simulink model "Modelo_nolineal_5GDL_COMPLETO_2022"  (R2021b)
settings: Solver=VariableStepAuto  StartTime=0.0  StopTime=5  FixedStep=T  RelTol=1e-3
values from neighbouring files (symbols this model uses):
  g = 9.81    [main.m]
undefined symbols (not defined in the file or in its folder): AG0, k1, k2, k3, l1, l2, l3, p1, p2, pod, ROTX_0, ROTY_0, ROTZ_0, y_ini, z_ini
settings Model: Creator=EDMAOR  LastModifiedBy=emate
settings SolverCC: AlgebraicLoopSolver=TrustRegion
settings DebuggingCC: SFMachineParentedDataDiag=warning
settings SFSimCC: CustomCodeUndefinedFunction=UseInterfaceOnly

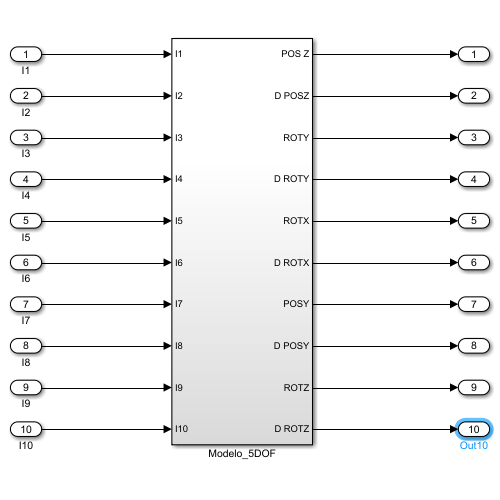
[thumbnail: Simulink's stored preview of the top-level diagram]
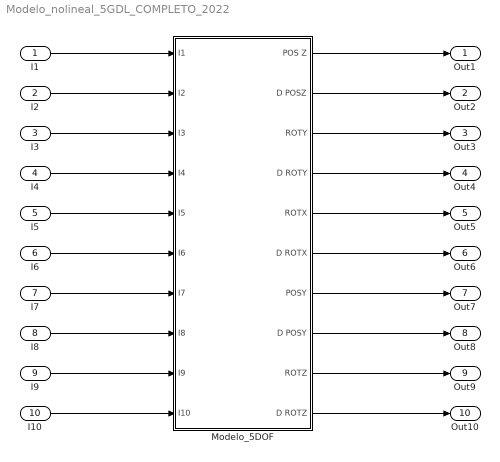
== system Modelo_nolineal_5GDL_COMPLETO_2022 ==
  I1 : Inport
  I2 : Inport  Port=2
  I3 : Inport  Port=3
  I4 : Inport  Port=4
  I5 : Inport  Port=5
  I6 : Inport  Port=6
  I7 : Inport  Port=7
  I8 : Inport  Port=8
  I9 : Inport  Port=9
  I10 : Inport  Port=10
  Modelo_5DOF : Subsystem
  Out1 : Outport
  Out2 : Outport  Port=2
  Out3 : Outport  Port=3
  Out4 : Outport  Port=4
  Out5 : Outport  Port=5
  Out6 : Outport  Port=6
  Out7 : Outport  Port=7
  Out8 : Outport  Port=8
  Out9 : Outport  Port=9
  Out10 : Outport  Port=10
  wires:
  Modelo_5DOF/1(POS Z) -> Out1/1
  I1/1 -> Modelo_5DOF/1(I1)
  I2/1 -> Modelo_5DOF/2(I2)
  I3/1 -> Modelo_5DOF/3(I3)
  I4/1 -> Modelo_5DOF/4(I4)
  I5/1 -> Modelo_5DOF/5(I5)
  I6/1 -> Modelo_5DOF/6(I6)
  Modelo_5DOF/2(D POSZ) -> Out2/1
  Modelo_5DOF/3(ROTY) -> Out3/1
  Modelo_5DOF/4(D ROTY) -> Out4/1
  Modelo_5DOF/5(ROTX) -> Out5/1
  Modelo_5DOF/6(D ROTX) -> Out6/1
  I7/1 -> Modelo_5DOF/7(I7)
  I8/1 -> Modelo_5DOF/8(I8)
  I9/1 -> Modelo_5DOF/9(I9)
  I10/1 -> Modelo_5DOF/10(I10)
  Modelo_5DOF/7(POSY) -> Out7/1
  Modelo_5DOF/8(D POSY) -> Out8/1
  Modelo_5DOF/9(ROTZ) -> Out9/1
  Modelo_5DOF/10(D ROTZ) -> Out10/1

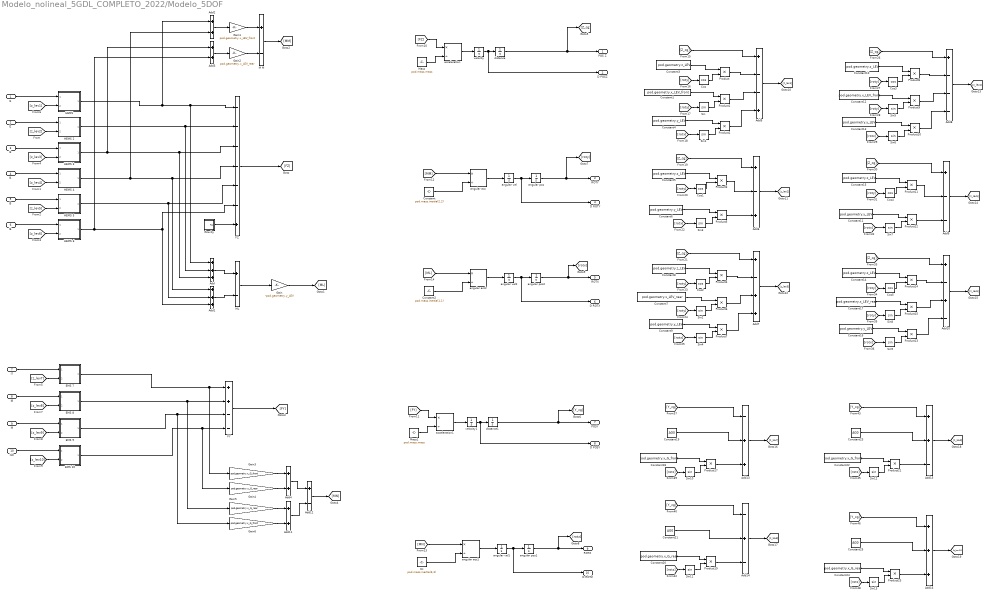
== system Modelo_nolineal_5GDL_COMPLETO_2022/Modelo_5DOF ==
  I1 : Inport
  I2 : Inport  Port=2
  I3 : Inport  Port=3
  I4 : Inport  Port=4
  I5 : Inport  Port=5
  I6 : Inport  Port=6
  I7 : Inport  Port=7
  I8 : Inport  Port=8
  I9 : Inport  Port=9
  I10 : Inport  Port=10
  Add : Sum  Inputs=+++
  Add1 : Sum  Inputs=+++
  Add10 : Sum  Inputs=+-+-
  Add{2..4,11} (4 alike) : Sum
  Add12 : Sum  Inputs=+-
  Add13 : Sum  Inputs=-++
  Add14 : Sum  Inputs=-+-
  Add15 : Sum  Inputs=++-
  Add16 : Sum  Inputs=+++
  Add5 : Sum  Inputs=+--+
  Add6 : Sum  Inputs=+-+
  Add7 : Sum  Inputs=+-++
  Add8 : Sum  Inputs=+---
  Add9 : Sum  Inputs=+--
  Constant : Constant  Value=pod.mass.inertia(2,2)
  Constant1 : Constant  Value=pod.geometry.x_LEV_front
  Constant{3,5,8,10,14..15} (6 alike) : Constant  Value=pod.geometry.z_LEV
  Constant{4,6,9,11,13,16} (6 alike) : Constant  Value=pod.geometry.y_LEV
  Constant12 : Constant  Value=pod.geometry.x_LEV_front
  Constant17 : Constant  Value=pod.geometry.x_LEV_rear
  Constant18 : Constant  Value=pod.geometry.x_G_front
  Constant{19,21,23,25} (4 alike) : Constant  Value=AG0
  Constant2 : Constant  Value=pod.mass.inertia(1,1)
  Constant20 : Constant  Value=pod.geometry.x_G_rear
  Constant22 : Constant  Value=pod.geometry.x_G_front
  Constant24 : Constant  Value=pod.geometry.x_G_rear
  Constant7 : Constant  Value=pod.geometry.x_LEV_rear
  Cos{,1..5} (6 alike) : Trigonometry  Operator=cos
  EMS 10 : Subsystem
  EMS 7 : Subsystem
  EMS 8 : Subsystem
  EMS 9 : Subsystem
  FY : Sum  Inputs=++--
  FZ : Sum  Inputs=------+
  Gain : Gain  Gain=-pod.geometry.y_LEV
  Gain1 : Gain  Gain=pod.geometry.x_LEV_front
  Gain2 : Gain  Gain=pod.geometry.x_LEV_rear
  Gain3 : Gain  Gain=pod.geometry.x_G_front
  Gain4 : Gain  Gain=pod.geometry.x_G_rear
  Gain5 : Gain  Gain=pod.geometry.x_G_rear
  Gain6 : Gain  Gain=pod.geometry.x_G_front
  Gravity : Subsystem
  "HEMS " : Subsystem
  HEMS 2 : Subsystem
  HEMS 3 : Subsystem
  HEMS 4 : Subsystem
  HEMS 5 : Subsystem
  HEMS 6 : Subsystem
  Izz : Constant  Value=pod.mass.inertia(3,3)
  M M : Sum  Inputs=+-
  ML : Sum  Inputs=+-
  Mass : Constant  Value=pod.mass.mass
  Mass1 : Constant  Value=pod.mass.mass
  Product{,1..15,17,19,21,23} (20 alike) : Product
  Sin{,1..13} (14 alike) : Trigonometry
  acceleration : Product  Inputs=*/
  acceleration1 : Product  Inputs=*/
  angular acc : Product  Inputs=*/
  angular acc1 : Product  Inputs=*/
  angular acc2 : Product  Inputs=*/
  angular pos : Integrator  InitialCondition=ROTY_0
  angular pos1 : Integrator  InitialCondition=ROTZ_0
  angular pos2 : Integrator  InitialCondition=ROTX_0
  angular vel : Integrator
  angular vel1 : Integrator
  angular vel2 : Integrator
  distance : Integrator  InitialCondition=z_ini
  distance1 : Integrator  InitialCondition=y_ini
  velocity : Integrator
  velocity1 : Integrator
  POS Z : Outport  VectorParamsAs1DForOutWhenUnconnected=off
  D POSZ : Outport  Port=2  VectorParamsAs1DForOutWhenUnconnected=off
  ROTY : Outport  Port=3  VectorParamsAs1DForOutWhenUnconnected=off
  D ROTY : Outport  Port=4  VectorParamsAs1DForOutWhenUnconnected=off
  ROTX : Outport  Port=5  VectorParamsAs1DForOutWhenUnconnected=off
  D ROTX : Outport  Port=6  VectorParamsAs1DForOutWhenUnconnected=off
  POSY : Outport  Port=7  VectorParamsAs1DForOutWhenUnconnected=off
  D POSY : Outport  Port=8  VectorParamsAs1DForOutWhenUnconnected=off
  ROTZ : Outport  Port=9  VectorParamsAs1DForOutWhenUnconnected=off
  D ROTZ : Outport  Port=10  VectorParamsAs1DForOutWhenUnconnected=off
  wires:
  acceleration/1 -> velocity/1
  velocity/1 -> D POSZ/1, distance/1
  distance/1 -> [Z_cg], POS Z/1
  I1/1 -> "HEMS "/1(current 1)
  I2/1 -> HEMS 2/1(current 2)
  I3/1 -> HEMS 3/1(current 3)
  "HEMS "/1(HEMS 1) -> Add/1, FZ/1, Add2/1
  HEMS 2/1(HEMS 2) -> Add/2, FZ/2
  HEMS 3/1(HEMS 3) -> Add/3, FZ/3, Add3/1
  Mass/1 -> acceleration/2
  [z_lev2] -> HEMS 2/2(distance 2)
  [z_lev3] -> HEMS 3/2(distance 3)
  [z_lev1] -> "HEMS "/2(distance 1)
  I4/1 -> HEMS 4/1(current 4)
  I5/1 -> HEMS 5/1(current 5)
  I6/1 -> HEMS 6/1(current 6)
  [z_lev4] -> HEMS 4/2(distance 4)
  [z_lev5] -> HEMS 5/2(distance 5)
  [z_lev6] -> HEMS 6/2(distance 6)
  HEMS 4/1(HEMS 4) -> Add1/1, FZ/4, Add2/2
  HEMS 5/1(HEMS 5) -> Add1/2, FZ/5
  HEMS 6/1(HEMS 6) -> Add1/3, FZ/6, Add3/2
  Gravity/1(Fg) -> FZ/7
  FZ/1 -> [FZ]
  ML/1 -> Gain/1
  Add1/1 -> ML/2
  Add/1 -> ML/1
  M M/1 -> [MM]
  Add2/1 -> Gain1/1
  Add3/1 -> Gain2/1
  Gain/1 -> [ML]
  [FZ] -> acceleration/1
  angular vel/1 -> D ROTY/1, angular pos/1
  angular pos/1 -> [roty], ROTY/1
  angular acc/1 -> angular vel/1
  [MM] -> angular acc/1
  Constant/1 -> angular acc/2
  angular pos2/1 -> [rotx], ROTX/1
  [ML] -> angular acc2/1
  angular vel2/1 -> angular pos2/1, D ROTX/1
  Constant2/1 -> angular acc2/2
  angular acc2/1 -> angular vel2/1
  [Z_cg] -> Add5/1
  Constant3/1 -> Product/1
  Cos/1 -> Product/2
  [roty] -> Cos/1
  Product/1 -> Add5/2
  [roty] -> Sin/1
  Sin/1 -> Product1/2
  Constant1/1 -> Product1/1
  Product1/1 -> Add5/3
  Constant4/1 -> Product2/1
  Sin1/1 -> Product2/2
  [rotx] -> Sin1/1
  Product2/1 -> Add5/4
  Add5/1 -> [z_lev1]
  Add6/1 -> [z_lev2]
  [rotx] -> Sin3/1
  Sin3/1 -> Product5/2
  Constant6/1 -> Product5/1
  Product3/1 -> Add6/2
  [roty] -> Cos1/1
  Cos1/1 -> Product3/2
  Constant5/1 -> Product3/1
  [Z_cg] -> Add6/1
  Product5/1 -> Add6/3
  Add7/1 -> [z_lev3]
  Product7/1 -> Add7/4
  [rotx] -> Sin4/1
  Sin4/1 -> Product7/2
  Constant9/1 -> Product7/1
  Product6/1 -> Add7/3
  Constant7/1 -> Product6/1
  Sin2/1 -> Product6/2
  [roty] -> Sin2/1
  Product4/1 -> Add7/2
  [roty] -> Cos2/1
  Cos2/1 -> Product4/2
  Constant8/1 -> Product4/1
  [Z_cg] -> Add7/1
  [Z_cg] -> Add8/1
  Constant10/1 -> Product8/1
  Cos3/1 -> Product8/2
  [roty] -> Cos3/1
  Product8/1 -> Add8/2
  [roty] -> Sin5/1
  Sin5/1 -> Product9/2
  Constant12/1 -> Product9/1
  Product9/1 -> Add8/3
  Constant13/1 -> Product10/1
  Sin6/1 -> Product10/2
  [rotx] -> Sin6/1
  Product10/1 -> Add8/4
  Add8/1 -> [z_lev4]
  Product12/1 -> Add9/3
  [Z_cg] -> Add9/1
  Constant15/1 -> Product11/1
  Cos4/1 -> Product11/2
  [roty] -> Cos4/1
  Product11/1 -> Add9/2
  Constant11/1 -> Product12/1
  Sin7/1 -> Product12/2
  [rotx] -> Sin7/1
  Add9/1 -> [z_lev5]
  Add10/1 -> [z_lev6]
  Product13/1 -> Add10/4
  [rotx] -> Sin9/1
  Sin9/1 -> Product13/2
  Constant16/1 -> Product13/1
  Product15/1 -> Add10/3
  Constant17/1 -> Product15/1
  Sin8/1 -> Product15/2
  [roty] -> Sin8/1
  Product14/1 -> Add10/2
  [roty] -> Cos5/1
  Cos5/1 -> Product14/2
  Constant14/1 -> Product14/1
  [Z_cg] -> Add10/1
  Gain1/1 -> M M/1
  Gain2/1 -> M M/2
  [z_lev10] -> EMS 10/2(distance 10)
  FY/1 -> [FY]
  EMS 10/1(EMS 10) -> Gain4/1, FY/4
  I9/1 -> EMS 9/1(current 9)
  EMS 8/1(EMS 8) -> Gain5/1, FY/2
  EMS 9/1(EMS 9) -> Gain6/1, FY/3
  EMS 7/1(EMS 7) -> Gain3/1, FY/1
  I8/1 -> EMS 8/1(current 8)
  Add11/1 -> Add12/2
  Add12/1 -> [MN]
  [z_lev7] -> EMS 7/2(distance 7)
  I7/1 -> EMS 7/1(current 7)
  Gain6/1 -> Add11/2
  Gain5/1 -> Add11/1
  I10/1 -> EMS 10/1(current 10)
  [z_lev8] -> EMS 8/2(distance 8)
  Gain3/1 -> Add4/1
  Gain4/1 -> Add4/2
  [z_lev9] -> EMS 9/2(distance 9)
  Add4/1 -> Add12/1
  distance1/1 -> [Y_cg], POSY/1
  angular vel1/1 -> D ROTZ/1, angular pos1/1
  Mass1/1 -> acceleration1/2
  [FY] -> acceleration1/1
  angular acc1/1 -> angular vel1/1
  Izz/1 -> angular acc1/2
  velocity1/1 -> distance1/1, D POSY/1
  angular pos1/1 -> [rotz], ROTZ/1
  acceleration1/1 -> velocity1/1
  [MN] -> angular acc1/1
  Sin11/1 -> Product19/2
  Product19/1 -> Add14/3
  [Y_cg] -> Add14/1
  [Y_cg] -> Add13/1
  Constant18/1 -> Product17/1
  Product17/1 -> Add13/3
  Constant19/1 -> Add13/2
  Add13/1 -> [z_lev7]
  [rotz] -> Sin10/1
  Constant20/1 -> Product19/1
  Sin10/1 -> Product17/2
  Constant21/1 -> Add14/2
  [rotz] -> Sin11/1
  Add14/1 -> [z_lev8]
  Constant25/1 -> Add16/2
  Constant23/1 -> Add15/2
  [Y_cg] -> Add15/1
  Constant22/1 -> Product21/1
  [rotz] -> Sin13/1
  [Y_cg] -> Add16/1
  Add16/1 -> [z_lev10]
  Product21/1 -> Add15/3
  Sin13/1 -> Product23/2
  [rotz] -> Sin12/1
  Add15/1 -> [z_lev9]
  Constant24/1 -> Product23/1
  Sin12/1 -> Product21/2
  Product23/1 -> Add16/3

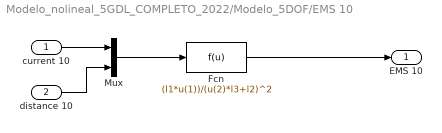
== system Modelo_nolineal_5GDL_COMPLETO_2022/Modelo_5DOF/EMS 10 ==
  current 10 : Inport
  distance 10 : Inport  Port=2
  Fcn : Fcn  Expr=(l1*u(1))/(u(2)*l3+l2)^2
  Mux : Mux  Inputs=2
  EMS 10 : Outport  VectorParamsAs1DForOutWhenUnconnected=off
  wires:
  Fcn/1 -> EMS 10/1
  Mux/1 -> Fcn/1
  distance 10/1 -> Mux/2
  current 10/1 -> Mux/1

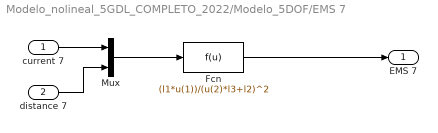
== system Modelo_nolineal_5GDL_COMPLETO_2022/Modelo_5DOF/EMS 7 ==
  current 7 : Inport
  distance 7 : Inport  Port=2
  Fcn : Fcn  Expr=(l1*u(1))/(u(2)*l3+l2)^2
  Mux : Mux  Inputs=2
  EMS 7 : Outport  VectorParamsAs1DForOutWhenUnconnected=off
  wires:
  current 7/1 -> Mux/1
  distance 7/1 -> Mux/2
  Mux/1 -> Fcn/1
  Fcn/1 -> EMS 7/1

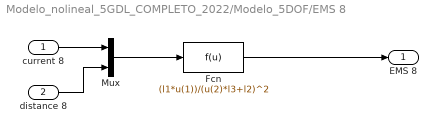
== system Modelo_nolineal_5GDL_COMPLETO_2022/Modelo_5DOF/EMS 8 ==
  current 8 : Inport
  distance 8 : Inport  Port=2
  Fcn : Fcn  Expr=(l1*u(1))/(u(2)*l3+l2)^2
  Mux : Mux  Inputs=2
  EMS 8 : Outport  VectorParamsAs1DForOutWhenUnconnected=off
  wires:
  Fcn/1 -> EMS 8/1
  Mux/1 -> Fcn/1
  distance 8/1 -> Mux/2
  current 8/1 -> Mux/1

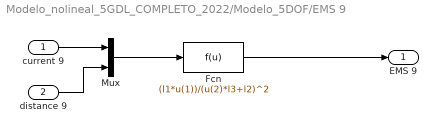
== system Modelo_nolineal_5GDL_COMPLETO_2022/Modelo_5DOF/EMS 9 ==
  current 9 : Inport
  distance 9 : Inport  Port=2
  Fcn : Fcn  Expr=(l1*u(1))/(u(2)*l3+l2)^2
  Mux : Mux  Inputs=2
  EMS 9 : Outport  VectorParamsAs1DForOutWhenUnconnected=off
  wires:
  current 9/1 -> Mux/1
  distance 9/1 -> Mux/2
  Mux/1 -> Fcn/1
  Fcn/1 -> EMS 9/1

== system Modelo_nolineal_5GDL_COMPLETO_2022/Modelo_5DOF/Gravity ==
  Fgrav : Subsystem
  Mass : Constant  Value=pod.mass.mass
  gravity : Constant  Value=g
  Fg : Outport
  wires:
  Fgrav/1(Fg) -> Fg/1
  gravity/1 -> Fgrav/1(gravity)
  Mass/1 -> Fgrav/2(mass)

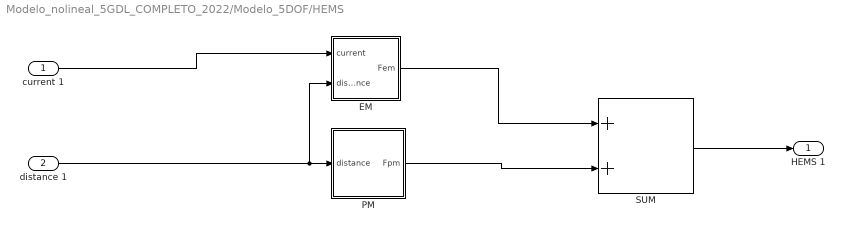
== system Modelo_nolineal_5GDL_COMPLETO_2022/Modelo_5DOF/HEMS  ==
  current 1 : Inport
  distance 1 : Inport  Port=2
  EM : Subsystem
  PM : Subsystem
  SUM : Sum
  HEMS 1 : Outport  VectorParamsAs1DForOutWhenUnconnected=off
  wires:
  PM/1(Fpm) -> SUM/2
  distance 1/1 -> EM/2(distance), PM/1(distance)
  EM/1(Fem) -> SUM/1
  current 1/1 -> EM/1(current)
  SUM/1 -> HEMS 1/1

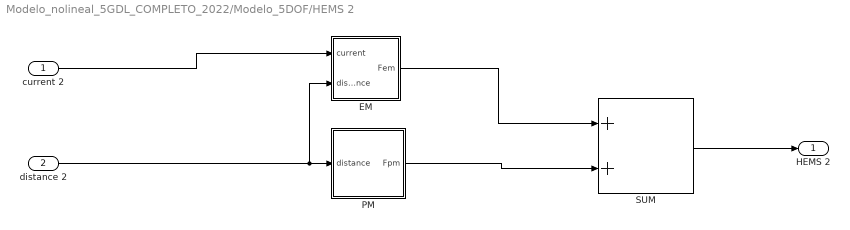
== system Modelo_nolineal_5GDL_COMPLETO_2022/Modelo_5DOF/HEMS 2 ==
  current 2 : Inport
  distance 2 : Inport  Port=2
  EM : Subsystem
  PM : Subsystem
  SUM : Sum
  HEMS 2 : Outport  VectorParamsAs1DForOutWhenUnconnected=off
  wires:
  SUM/1 -> HEMS 2/1
  current 2/1 -> EM/1(current)
  EM/1(Fem) -> SUM/1
  distance 2/1 -> PM/1(distance), EM/2(distance)
  PM/1(Fpm) -> SUM/2

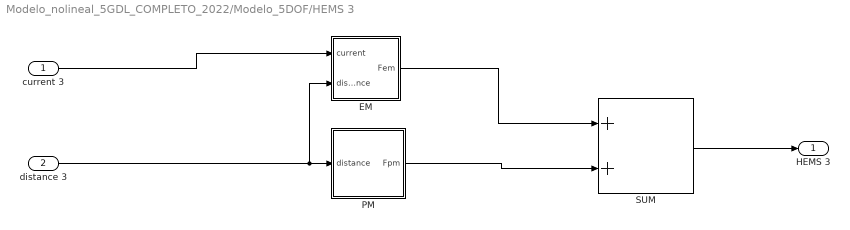
== system Modelo_nolineal_5GDL_COMPLETO_2022/Modelo_5DOF/HEMS 3 ==
  current 3 : Inport
  distance 3 : Inport  Port=2
  EM : Subsystem
  PM : Subsystem
  SUM : Sum
  HEMS 3 : Outport  VectorParamsAs1DForOutWhenUnconnected=off
  wires:
  PM/1(Fpm) -> SUM/2
  distance 3/1 -> EM/2(distance), PM/1(distance)
  EM/1(Fem) -> SUM/1
  current 3/1 -> EM/1(current)
  SUM/1 -> HEMS 3/1

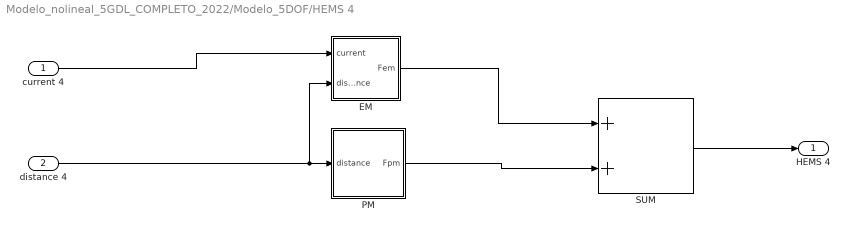
== system Modelo_nolineal_5GDL_COMPLETO_2022/Modelo_5DOF/HEMS 4 ==
  current 4 : Inport
  distance 4 : Inport  Port=2
  EM : Subsystem
  PM : Subsystem
  SUM : Sum
  HEMS 4 : Outport  VectorParamsAs1DForOutWhenUnconnected=off
  wires:
  SUM/1 -> HEMS 4/1
  current 4/1 -> EM/1(current)
  EM/1(Fem) -> SUM/1
  distance 4/1 -> PM/1(distance), EM/2(distance)
  PM/1(Fpm) -> SUM/2

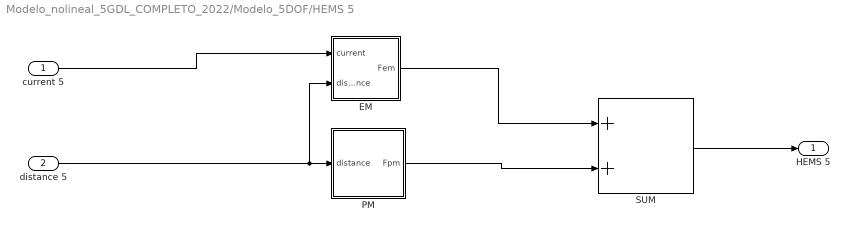
== system Modelo_nolineal_5GDL_COMPLETO_2022/Modelo_5DOF/HEMS 5 ==
  current 5 : Inport
  distance 5 : Inport  Port=2
  EM : Subsystem
  PM : Subsystem
  SUM : Sum
  HEMS 5 : Outport  VectorParamsAs1DForOutWhenUnconnected=off
  wires:
  PM/1(Fpm) -> SUM/2
  distance 5/1 -> EM/2(distance), PM/1(distance)
  EM/1(Fem) -> SUM/1
  current 5/1 -> EM/1(current)
  SUM/1 -> HEMS 5/1

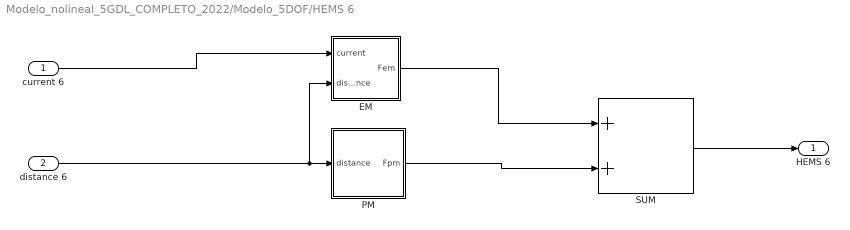
== system Modelo_nolineal_5GDL_COMPLETO_2022/Modelo_5DOF/HEMS 6 ==
  current 6 : Inport
  distance 6 : Inport  Port=2
  EM : Subsystem
  PM : Subsystem
  SUM : Sum
  HEMS 6 : Outport  VectorParamsAs1DForOutWhenUnconnected=off
  wires:
  SUM/1 -> HEMS 6/1
  current 6/1 -> EM/1(current)
  EM/1(Fem) -> SUM/1
  distance 6/1 -> PM/1(distance), EM/2(distance)
  PM/1(Fpm) -> SUM/2

== system Modelo_nolineal_5GDL_COMPLETO_2022/Modelo_5DOF/Gravity/Fgrav ==
  gravity : Inport
  mass : Inport  Port=2
  Product : Product
  Fg : Outport  VectorParamsAs1DForOutWhenUnconnected=off
  wires:
  Product/1 -> Fg/1
  gravity/1 -> Product/1
  mass/1 -> Product/2

== system Modelo_nolineal_5GDL_COMPLETO_2022/Modelo_5DOF/HEMS /EM ==
  current : Inport
  distance : Inport  Port=2
  Fcn : Fcn  Expr=(k1*u(1))/(u(2)*k3-k2)^2
  Mux : Mux  Inputs=2
  Fem : Outport  VectorParamsAs1DForOutWhenUnconnected=off
  wires:
  current/1 -> Mux/1
  distance/1 -> Mux/2
  Mux/1 -> Fcn/1
  Fcn/1 -> Fem/1

== system Modelo_nolineal_5GDL_COMPLETO_2022/Modelo_5DOF/HEMS /PM ==
  distance : Inport
  Fcn1 : Fcn  Expr=p1/(p2+u(1))^2
  Fpm : Outport  VectorParamsAs1DForOutWhenUnconnected=off
  wires:
  distance/1 -> Fcn1/1
  Fcn1/1 -> Fpm/1

== system Modelo_nolineal_5GDL_COMPLETO_2022/Modelo_5DOF/HEMS 2/EM ==
  current : Inport
  distance : Inport  Port=2
  Fcn : Fcn  Expr=(k1*u(1))/(u(2)*k3-k2)^2
  Mux : Mux  Inputs=2
  Fem : Outport  VectorParamsAs1DForOutWhenUnconnected=off
  wires:
  Fcn/1 -> Fem/1
  Mux/1 -> Fcn/1
  distance/1 -> Mux/2
  current/1 -> Mux/1

== system Modelo_nolineal_5GDL_COMPLETO_2022/Modelo_5DOF/HEMS 2/PM ==
  distance : Inport
  Fcn1 : Fcn  Expr=p1/(p2+u(1))^2
  Fpm : Outport  VectorParamsAs1DForOutWhenUnconnected=off
  wires:
  Fcn1/1 -> Fpm/1
  distance/1 -> Fcn1/1

== system Modelo_nolineal_5GDL_COMPLETO_2022/Modelo_5DOF/HEMS 3/EM ==
  current : Inport
  distance : Inport  Port=2
  Fcn : Fcn  Expr=(k1*u(1))/(u(2)*k3-k2)^2
  Mux : Mux  Inputs=2
  Fem : Outport  VectorParamsAs1DForOutWhenUnconnected=off
  wires:
  current/1 -> Mux/1
  distance/1 -> Mux/2
  Mux/1 -> Fcn/1
  Fcn/1 -> Fem/1

== system Modelo_nolineal_5GDL_COMPLETO_2022/Modelo_5DOF/HEMS 3/PM ==
  distance : Inport
  Fcn1 : Fcn  Expr=p1/(p2+u(1))^2
  Fpm : Outport  VectorParamsAs1DForOutWhenUnconnected=off
  wires:
  distance/1 -> Fcn1/1
  Fcn1/1 -> Fpm/1

== system Modelo_nolineal_5GDL_COMPLETO_2022/Modelo_5DOF/HEMS 4/EM ==
  current : Inport
  distance : Inport  Port=2
  Fcn : Fcn  Expr=(k1*u(1))/(u(2)*k3-k2)^2
  Mux : Mux  Inputs=2
  Fem : Outport  VectorParamsAs1DForOutWhenUnconnected=off
  wires:
  Fcn/1 -> Fem/1
  Mux/1 -> Fcn/1
  distance/1 -> Mux/2
  current/1 -> Mux/1

== system Modelo_nolineal_5GDL_COMPLETO_2022/Modelo_5DOF/HEMS 4/PM ==
  distance : Inport
  Fcn1 : Fcn  Expr=p1/(p2+u(1))^2
  Fpm : Outport  VectorParamsAs1DForOutWhenUnconnected=off
  wires:
  Fcn1/1 -> Fpm/1
  distance/1 -> Fcn1/1

== system Modelo_nolineal_5GDL_COMPLETO_2022/Modelo_5DOF/HEMS 5/EM ==
  current : Inport
  distance : Inport  Port=2
  Fcn : Fcn  Expr=(k1*u(1))/(u(2)*k3-k2)^2
  Mux : Mux  Inputs=2
  Fem : Outport  VectorParamsAs1DForOutWhenUnconnected=off
  wires:
  current/1 -> Mux/1
  distance/1 -> Mux/2
  Mux/1 -> Fcn/1
  Fcn/1 -> Fem/1

== system Modelo_nolineal_5GDL_COMPLETO_2022/Modelo_5DOF/HEMS 5/PM ==
  distance : Inport
  Fcn1 : Fcn  Expr=p1/(p2+u(1))^2
  Fpm : Outport  VectorParamsAs1DForOutWhenUnconnected=off
  wires:
  distance/1 -> Fcn1/1
  Fcn1/1 -> Fpm/1

== system Modelo_nolineal_5GDL_COMPLETO_2022/Modelo_5DOF/HEMS 6/EM ==
  current : Inport
  distance : Inport  Port=2
  Fcn : Fcn  Expr=(k1*u(1))/(u(2)*k3-k2)^2
  Mux : Mux  Inputs=2
  Fem : Outport  VectorParamsAs1DForOutWhenUnconnected=off
  wires:
  Fcn/1 -> Fem/1
  Mux/1 -> Fcn/1
  distance/1 -> Mux/2
  current/1 -> Mux/1

== system Modelo_nolineal_5GDL_COMPLETO_2022/Modelo_5DOF/HEMS 6/PM ==
  distance : Inport
  Fcn1 : Fcn  Expr=p1/(p2+u(1))^2
  Fpm : Outport  VectorParamsAs1DForOutWhenUnconnected=off
  wires:
  Fcn1/1 -> Fpm/1
  distance/1 -> Fcn1/1
